simulink model "esotest"  (R2018a)
settings: Solver=VariableStepAuto  StartTime=0.0  StopTime=10.0  RelTol=1e-3
settings Model: Creator=Ducted Fan  LastModifiedBy=Ducted Fan

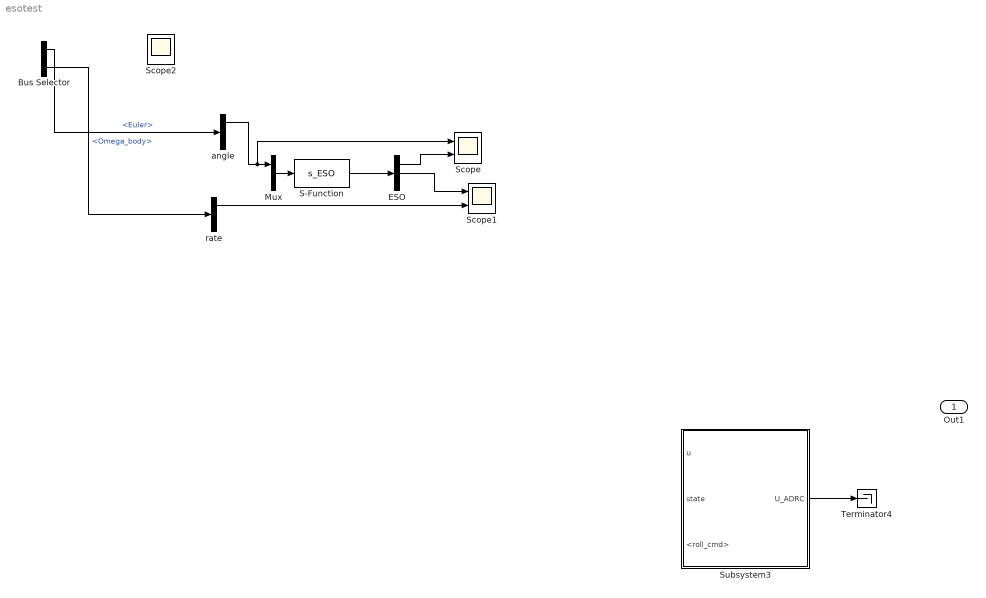
== system esotest ==
  Bus Selector : BusSelector  OutputSignals=Euler,Omega_body
  ESO : Demux  Outputs=3
  Mux : Mux  Inputs=2
  S-Function : S-Function  FunctionName=s_ESO  SFunctionDeploymentMode=off  EnableBusSupport=off
  Scope : Scope  NumInputPorts=2
  Scope1 : Scope  NumInputPorts=2
  Scope2 : Scope
  Subsystem3 : Subsystem
  Terminator4 : Terminator
  angle : Demux  Outputs=3
  rate : Demux  Outputs=3
  Out1 : Outport
  wires:
  ESO/1 -> Scope/2
  Bus Selector/1 -> angle/1  "<Euler>"
  ESO/2 -> Scope1/1
  ? -> Bus Selector/1  "States"
  angle/1 -> Scope/1, Mux/1
  Bus Selector/2 -> rate/1  "<Omega_body>"
  S-Function/1 -> ESO/1
  rate/1 -> Scope1/2
  Mux/1 -> S-Function/1
  Subsystem3/1("U_ADRC ") -> Terminator4/1
  ? -> Subsystem3/3(<roll_cmd>)  "<roll_cmd>"
  ? -> Subsystem3/2(state)

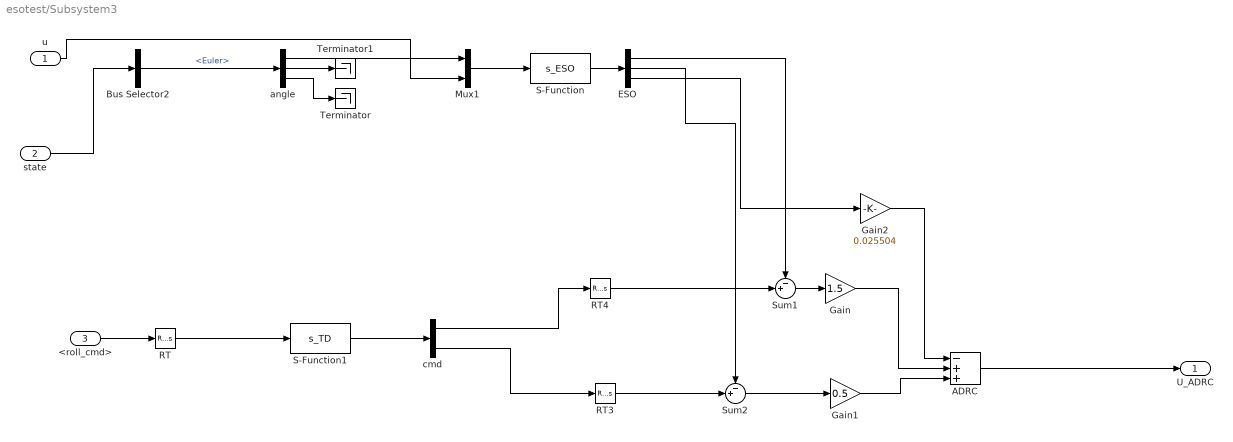
== system esotest/Subsystem3 ==
  "u " : Inport
  state : Inport  Port=2
  <roll_cmd> : Inport  Port=3
  ADRC : Sum  Inputs=-++
  Bus Selector2 : BusSelector  OutputSignals=Euler
  ESO : Demux  Outputs=3
  Gain : Gain  Gain=1.5
  Gain1 : Gain  Gain=0.5
  Gain2 : Gain  Gain=0.025504
  Mux1 : Mux  Inputs=2
  RT : RateTransition  OutPortSampleTime=0.05
  RT3 : RateTransition  OutPortSampleTime=0.01
  RT4 : RateTransition  OutPortSampleTime=0.01
  S-Function : S-Function  FunctionName=s_ESO  SFunctionDeploymentMode=off  EnableBusSupport=off
  S-Function1 : S-Function  FunctionName=s_TD  SFunctionDeploymentMode=off  EnableBusSupport=off
  Sum1 : Sum  Inputs=-+|
  Sum2 : Sum  Inputs=-+|
  Terminator : Terminator
  Terminator1 : Terminator
  angle : Demux  Outputs=3
  cmd : Demux  Outputs=2
  "U_ADRC " : Outport
  wires:
  cmd/2 -> RT3/1
  angle/1 -> Mux1/1
  S-Function/1 -> ESO/1
  ESO/2 -> Sum2/1
  Gain2/1 -> ADRC/1
  ESO/1 -> Sum1/1
  Mux1/1 -> S-Function/1
  <roll_cmd>/1 -> RT/1
  RT4/1 -> Sum1/2
  "u "/1 -> Mux1/2
  ESO/3 -> Gain2/1
  ADRC/1 -> "U_ADRC "/1
  Bus Selector2/1 -> angle/1  "<Euler>"
  Sum1/1 -> Gain/1
  Gain1/1 -> ADRC/3
  cmd/1 -> RT4/1
  Sum2/1 -> Gain1/1
  S-Function1/1 -> cmd/1
  RT3/1 -> Sum2/2
  angle/3 -> Terminator/1
  Gain/1 -> ADRC/2
  RT/1 -> S-Function1/1
  state/1 -> Bus Selector2/1
  angle/2 -> Terminator1/1
